simulink model "feng_rx_ct_pack"  (R2012b)
settings: Solver=FixedStepDiscrete  SolverMode=SingleTasking  StartTime=0.0  StopTime=30000  FixedStep=1  RelTol=1e-3
libraries: xbsIndex_r4 x1581, xps_library x3, casper_library_delays x2
(part 2 of 11)

== system feng_rx_ct_pack/gap_enforcer ==
  sync : Inport
  din : Inport  Port=2
  en : Inport  Port=3
  Concat : xbsIndex_r4/Concat  num_inputs=2  dbl_ovrd=off  block_type=concat
  Delay : xbsIndex_r4/Delay  rst=off  infoeditControl=Selection of Reset will increase slice count due to use of real FFs and instead of SRLs  en=off  latency=1  dbl_ovrd=off  reg_retiming=off  block_type=delay
  FIFO : xbsIndex_r4/FIFO  mem_type=Distributed RAM  performance_options=Standard_FIFO  infoedit1=Available only for V4, V5, V6, V7, K7, A7 and Zynq devices.  embedded_registers=off  depth=16  percent_nbits=2  rst=off  en=off  use_dcount=off  use_percent_full_port=off  use_almost_empty=off  almost_empty_thresh=2  use_almost_full=off  almost_full_thresh=14  dbl_ovrd=off  explicit_period=off  block_type=fifo
  Gateway Out{,1..7} (8 alike) : xbsIndex_r4/Gateway Out  inherit_from_input=off  hdl_port=on  timing_constraint=None  locs_specified=off  LOCs={}  UseAsDAC=off  DACChannel='1'  block_type=gatewayout
  Inverter : xbsIndex_r4/Inverter  en=off  latency=0  dbl_ovrd=off  block_type=inv
  Logical : xbsIndex_r4/Logical  logical_function=AND  inputs=2  en=off  latency=0  precision=Full  arith_type=Unsigned  n_bits=16  bin_pt=0  align_bp=on  dbl_ovrd=off  block_type=logical
  Scope : Scope  NumInputPorts=8
      settings: YMin=0~0~0~0~0~-1~0~-1  YMax=1~1~1~150~1~1~300~1
  Slice2 : xbsIndex_r4/Slice  nbits=1  boolean_output=off  mode=Two Bit Locations  bit1=-1  base1=MSB of Input  bit0=0  base0=LSB of Input  dbl_ovrd=off  block_type=slice
  Slice3 : xbsIndex_r4/Slice  nbits=1  boolean_output=on  mode=Upper Bit Location + Width  bit1=0  base1=MSB of Input  bit0=0  base0=LSB of Input  dbl_ovrd=off  block_type=slice
  Terminator1 : Terminator
  block_size : xbsIndex_r4/Constant  const=block_size  gui_display_data_type=Fixed-point  arith_type=Unsigned  n_bits=ceil(log2(block_size+gap_size))  bin_pt=0  preci_type=Single  exp_width=8  frac_width=24  explicit_period=on  period=1  equ=P=C  opselect=C  inp2=PCIN>>17  opr=+  inp1=P  carry=CIN  dbl_ovrd=off  block_type=constant
  data_count : xbsIndex_r4/Counter  cnt_type=Count Limited  cnt_to=block_size + gap_size  operation=Up  start_count=0  cnt_by_val=1  arith_type=Unsigned  n_bits=ceil(log2(block_size + gap_size))  bin_pt=0  load_pin=off  rst=on  en=on  explicit_period=on  period=1  dbl_ovrd=off  use_behavioral_HDL=off  implementation=Fabric  block_type=counter
  edge_detect1 : Subsystem  AncestorBlock=casper_library_misc/edge_detect  mask(edge_detect){edge=Rising, polarity=Active High, x_in=[0 0.08 0.08 0.16 0.16 0.24 0.24 0.32 0.32 0.4], y_in=[-1 -1  1  1  1  1  1  1  1  1], x_out=[0.6 0.68 0.68 0.76 0.76 0.84 0.84 0.92 0.92 1], y_out=[-1 -1  1  1 -1 -1 -1 -1 -1 -1]}
      mask prompts: edge "Edge Type"; polarity "Output Polarity"; x_in "Input X Positions"; y_in "Input Y Positions"; x_out "Output X Positions"; y_out "Output Y Positions"
      mask help: Output is active for one-cycle after each edge of the specified type (i.e. rising, falling or both).
      mask init:
      | edge_detect_init(gcb,...
      |     'edge',edge,...
      |     'polarity',polarity,...
      |     'x_in',x_in,...
      |     'x_out',x_out,...
      |     'y_in',y_in,...
      |     'y_out',y_out);
      | 
      | x_in_num=str2num(getfield(getfield(get_param(gcb,'UserData'),'parameters'),'x_in'));
      | x_out_num=str2num(getfield(getfield(get_param(gcb,'UserData'),'parameters'),'x_out'));
      | y_in_num=str2num(getfield(getfield(get_param(gcb,'UserData'),'parameters'),'y_in'));
      | y_out_num=str2num(getfield(getfield(get_param(gcb,'UserData'),'parameters'),'y_out'));
      settings: AttributesFormatString=|
      | rising edges
      | active high
      mask Help: Output is active for one-cycle after each edge of the specified type (i.e. rising, falling, or both).  Latency is zero.
      mask TypeOptions edge: Rising | Falling | Both
      mask TypeOptions polarity: Active High | Active Low
      mask Display:
      | plot(x_in_num,0.5+y_in_num*0.2);
      | plot(x_out_num,0.5+y_out_num*0.2);
  post_gap : xbsIndex_r4/Relational  mode=a<b  en=off  latency=0  dbl_ovrd=off  block_type=relational
  sync_out : Outport
  dout : Outport  Port=2
  dvalid : Outport  Port=3
  wires:
  edge_detect1/1(out) -> sync_out/1, Gateway Out5/1, data_count/1
  Logical/1 -> FIFO/3, Delay/1
  FIFO/2 -> Inverter/1
  FIFO/3 -> Terminator1/1
  post_gap/1 -> Gateway Out4/1, Logical/1
  Slice2/1 -> dout/1, Gateway Out6/1
  Inverter/1 -> Gateway Out2/1, data_count/2, Logical/2
  Slice3/1 -> edge_detect1/1(in)
  FIFO/1 -> Slice3/1, Slice2/1
  Concat/1 -> FIFO/1
  din/1 -> Concat/2
  Delay/1 -> dvalid/1, Gateway Out7/1
  en/1 -> FIFO/2, Gateway Out/1
  sync/1 -> Concat/1, Gateway Out1/1
  Gateway Out7/1 -> Scope/8
  Gateway Out6/1 -> Scope/7
  Gateway Out2/1 -> Scope/3
  Gateway Out3/1 -> Scope/4
  Gateway Out5/1 -> Scope/6
  Gateway Out4/1 -> Scope/5
  Gateway Out/1 -> Scope/1
  Gateway Out1/1 -> Scope/2
  block_size/1 -> post_gap/2
  data_count/1 -> Gateway Out3/1, post_gap/1

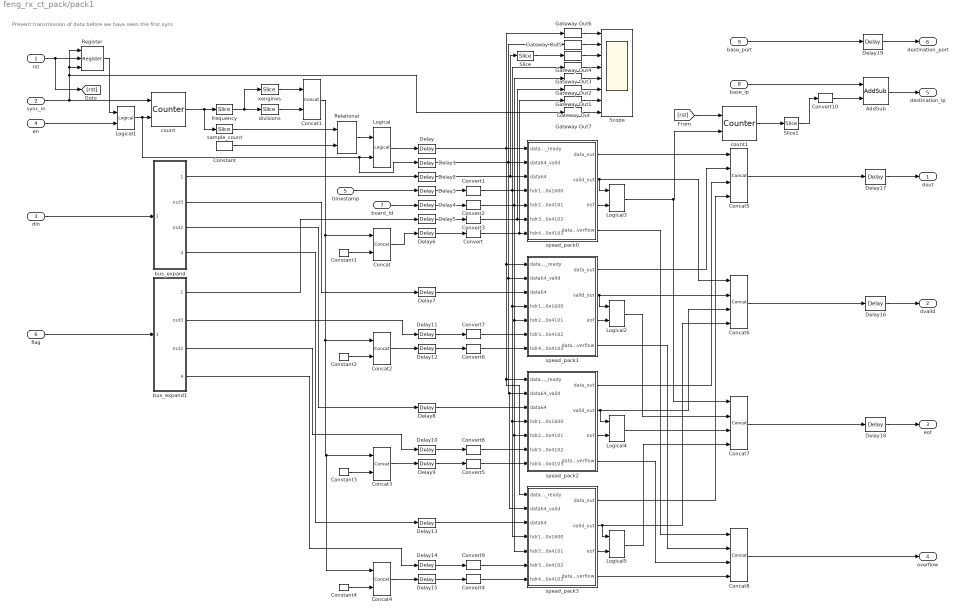
== system feng_rx_ct_pack/pack1 ==
  note: Prevent transmission of data
      | before we have seen the first
      | sync
  rst : Inport
  sync_in : Inport  Port=2
  din : Inport  Port=3
  en : Inport  Port=4
  timestamp : Inport  Port=5
  flag : Inport  Port=6
  board_id : Inport  Port=7
  base_ip : Inport  Port=8
  base_port : Inport  Port=9
  AddSub : xbsIndex_r4/AddSub  mode=Addition  use_carryin=off  use_carryout=off  en=off  latency=1  precision=User Defined  arith_type=Unsigned  n_bits=32  bin_pt=0  quantization=Truncate  overflow=Wrap  dbl_ovrd=off  use_behavioral_HDL=off  hw_selection=Fabric  pipelined=off  block_type=addsub
  Concat{,1..4} (5 alike) : xbsIndex_r4/Concat  num_inputs=2  dbl_ovrd=off  block_type=concat
  Concat{5..8} (4 alike) : xbsIndex_r4/Concat  num_inputs=4  dbl_ovrd=off  block_type=concat
  Constant : xbsIndex_r4/Constant  const=0  gui_display_data_type=Fixed-point  arith_type=Unsigned  n_bits=n_bits_packet - n_bits_inputs  bin_pt=0  preci_type=Single  exp_width=8  frac_width=24  explicit_period=on  period=1  equ=P=C  opselect=C  inp2=PCIN>>17  opr=+  inp1=P  carry=CIN  dbl_ovrd=off  block_type=constant
  Constant1 : xbsIndex_r4/Constant  const=0  gui_display_data_type=Fixed-point  arith_type=Unsigned  n_bits=2  bin_pt=0  preci_type=Single  exp_width=8  frac_width=24  explicit_period=on  period=1  equ=P=C  opselect=C  inp2=PCIN>>17  opr=+  inp1=P  carry=CIN  dbl_ovrd=off  block_type=constant
  Constant2 : xbsIndex_r4/Constant  const=1  gui_display_data_type=Fixed-point  arith_type=Unsigned  n_bits=2  bin_pt=0  preci_type=Single  exp_width=8  frac_width=24  explicit_period=on  period=1  equ=P=C  opselect=C  inp2=PCIN>>17  opr=+  inp1=P  carry=CIN  dbl_ovrd=off  block_type=constant
  Constant3 : xbsIndex_r4/Constant  const=2  gui_display_data_type=Fixed-point  arith_type=Unsigned  n_bits=2  bin_pt=0  preci_type=Single  exp_width=8  frac_width=24  explicit_period=on  period=1  equ=P=C  opselect=C  inp2=PCIN>>17  opr=+  inp1=P  carry=CIN  dbl_ovrd=off  block_type=constant
  Constant4 : xbsIndex_r4/Constant  const=3  gui_display_data_type=Fixed-point  arith_type=Unsigned  n_bits=2  bin_pt=0  preci_type=Single  exp_width=8  frac_width=24  explicit_period=on  period=1  equ=P=C  opselect=C  inp2=PCIN>>17  opr=+  inp1=P  carry=CIN  dbl_ovrd=off  block_type=constant
  Convert{,1..9} (10 alike) : xbsIndex_r4/Convert  gui_display_data_type=Fixed-point  arith_type=Unsigned  n_bits=48  bin_pt=0  float_type=Single  exp_bits=8  fraction_bits=24  quantization=Truncate  overflow=Wrap  en=off  latency=0  dbl_ovrd=off  pipeline=off  block_type=convert
  Convert10 : xbsIndex_r4/Convert  gui_display_data_type=Fixed-point  arith_type=Unsigned  n_bits=32  bin_pt=0  float_type=Single  exp_bits=8  fraction_bits=24  quantization=Truncate  overflow=Wrap  en=off  latency=0  dbl_ovrd=off  pipeline=off  block_type=convert
  Delay{,16..19} (5 alike) : xbsIndex_r4/Delay  rst=off  infoeditControl=Selection of Reset will increase slice count due to use of real FFs and instead of SRLs  en=off  latency=1  dbl_ovrd=off  reg_retiming=on  block_type=delay
  Delay{1..15} (15 alike) : xbsIndex_r4/Delay  rst=off  infoeditControl=Selection of Reset will increase slice count due to use of real FFs and instead of SRLs  en=off  latency=2  dbl_ovrd=off  reg_retiming=on  block_type=delay
  Gateway Out{,1..7} (8 alike) : xbsIndex_r4/Gateway Out  inherit_from_input=off  hdl_port=on  timing_constraint=None  locs_specified=off  LOCs={}  UseAsDAC=off  DACChannel='1'  block_type=gatewayout
  Logical{,1..5} (6 alike) : xbsIndex_r4/Logical  logical_function=AND  inputs=2  en=off  latency=0  precision=Full  arith_type=Unsigned  n_bits=16  bin_pt=0  align_bp=on  dbl_ovrd=off  block_type=logical
  Register : xbsIndex_r4/Register  init=0  rst=on  en=on  dbl_ovrd=off  block_type=register
  Relational : xbsIndex_r4/Relational  mode=a=b  en=off  latency=0  dbl_ovrd=off  block_type=relational
  Scope : Scope  NumInputPorts=8
      settings: YMin=-1~-1~832.2~3.11296e+06~-1~-1~26.6~-1  YMax=1~1~919.8~3.44064e+06~1~1~29.4~1  SaveName=ScopeData11
  Slice : xbsIndex_r4/Slice  nbits=16  boolean_output=off  mode=Upper Bit Location + Width  bit1=0  base1=MSB of Input  bit0=0  base0=LSB of Input  dbl_ovrd=off  block_type=slice
  Slice1 : xbsIndex_r4/Slice  nbits=n_bits_xengines - n_bits_xeng_per_ip  boolean_output=off  mode=Upper Bit Location + Width  bit1=0  base1=MSB of Input  bit0=0  base0=LSB of Input  dbl_ovrd=off  block_type=slice
  bus_expand : Subsystem  AncestorBlock=casper_library_flow_control/bus_expand  mask(bus_expand){mode=divisions of equal size, outputNum=4, outputWidth=64, outputBinaryPt=0, outputArithmeticType=0, show_format=off, outputToWorkspace=off, variablePrefix=out, outputToModelAsWell=on}
      mask prompts: outputNum "Number of outputs:"; outputWidth "Output width:"; outputBinaryPt "Output binary point position:"; outputArithmeticType "Output arithmetic type (ufix=0, fix=1, bool=2):"; show_format "Print format string?"; outputToWorkspace "Output to workspace?"; variablePrefix "Variable name prefix:"; outputToModelAsWell "Output to model as well?"
      mask help:
      | Expands a 'bus' made using a bus_create or Xilinx
      | concat block.
      | The input will be divided into the specified number
      | of outputs with the specified arithmetic types.
      | Divisions are made from most significant bit.
      mask init: same as feng_rx_ct_pack/bus_expand11
      settings: AttributesFormatString=4 outputs
      mask TypeOptions mode: divisions of equal size | divisions of arbitrary size
      mask Callback mode: bus_expand_callback();
      mask Callback outputWidth: bus_expand_callback();
      mask Callback outputToWorkspace: bus_expand_callback();
  bus_expand1 : Subsystem  AncestorBlock=casper_library_flow_control/bus_expand  mask(bus_expand){mode=divisions of equal size, outputNum=4, outputWidth=1, outputBinaryPt=0, outputArithmeticType=0, show_format=off, outputToWorkspace=off, variablePrefix=out, outputToModelAsWell=on}
      mask prompts: outputNum "Number of outputs:"; outputWidth "Output width:"; outputBinaryPt "Output binary point position:"; outputArithmeticType "Output arithmetic type (ufix=0, fix=1, bool=2):"; show_format "Print format string?"; outputToWorkspace "Output to workspace?"; variablePrefix "Variable name prefix:"; outputToModelAsWell "Output to model as well?"
      mask help:
      | Expands a 'bus' made using a bus_create or Xilinx
      | concat block.
      | The input will be divided into the specified number
      | of outputs with the specified arithmetic types.
      | Divisions are made from most significant bit.
      mask init: same as feng_rx_ct_pack/bus_expand11
      settings: AttributesFormatString=4 outputs
      mask TypeOptions mode: divisions of equal size | divisions of arbitrary size
      mask Callback mode: bus_expand_callback();
      mask Callback outputWidth: bus_expand_callback();
      mask Callback outputToWorkspace: bus_expand_callback();
  count : xbsIndex_r4/Counter  cnt_type=Free Running  cnt_to=Inf  operation=Up  start_count=0  cnt_by_val=1  arith_type=Unsigned  n_bits=n_bits_frequencies + n_bits_packet - n_bits_inputs  bin_pt=0  load_pin=off  rst=on  en=on  explicit_period=on  period=1  dbl_ovrd=off  use_behavioral_HDL=off  implementation=Fabric  block_type=counter
  count1 : xbsIndex_r4/Counter  cnt_type=Free Running  cnt_to=Inf  operation=Up  start_count=0  cnt_by_val=1  arith_type=Unsigned  n_bits=n_bits_xengines  bin_pt=0  load_pin=off  rst=on  en=on  explicit_period=on  period=1  dbl_ovrd=off  use_behavioral_HDL=off  implementation=Fabric  block_type=counter
  divisions : xbsIndex_r4/Slice  nbits=n_bits_frequencies - n_bits_xengines  boolean_output=off  mode=Upper Bit Location + Width  bit1=0  base1=MSB of Input  bit0=0  base0=LSB of Input  dbl_ovrd=off  block_type=slice
  frequency : xbsIndex_r4/Slice  nbits=n_bits_frequencies  boolean_output=off  mode=Upper Bit Location + Width  bit1=0  base1=MSB of Input  bit0=0  base0=LSB of Input  dbl_ovrd=off  block_type=slice
  sample_count : xbsIndex_r4/Slice  nbits=n_bits_packet - n_bits_inputs  boolean_output=off  mode=Lower Bit Location + Width  bit1=0  base1=MSB of Input  bit0=0  base0=LSB of Input  dbl_ovrd=off  block_type=slice
  spead_pack0 : Subsystem  Tag=casper:spead_pack  AncestorBlock=casper_library_communications/spead_pack  mask(pkt_pack_mask){payload_length=2^(n_bits_packet - n_bits_inputs), header_ids=hex2dec({'1600', '4101', '4102', '4103'}), spead_msw=64, spead_lsw=48, spead_version=4}
      mask prompts: payload_length "Payload Length in 64-bit words"; header_ids "SPEAD header IDs (decimal)"; spead_msw "SPEAD Flavour (MSw)"; spead_lsw "SPEAD Flavour (LSw)"; spead_version "SPEAD version"
      mask help:
      | This block generates SPEAD-compliant packets from a datastream.
      |
      | Packets are created with a fixed header followed by a number of 64-bit items.
      |
      | Requires a 64-bit data stream.
      |
      | See the documentation for further details.
      mask init:
      | spead_pack_init(gcb, header_ids)
  spead_pack1 : Subsystem  Tag=casper:spead_pack  AncestorBlock=casper_library_communications/spead_pack  mask(pkt_pack_mask){payload_length=2^(n_bits_packet - n_bits_inputs), header_ids=hex2dec({'1600', '4101', '4102', '4103'}), spead_msw=64, spead_lsw=48, spead_version=4}
      mask prompts: payload_length "Payload Length in 64-bit words"; header_ids "SPEAD header IDs (decimal)"; spead_msw "SPEAD Flavour (MSw)"; spead_lsw "SPEAD Flavour (LSw)"; spead_version "SPEAD version"
      mask help:
      | This block generates SPEAD-compliant packets from a datastream.
      |
      | Packets are created with a fixed header followed by a number of 64-bit items.
      |
      | Requires a 64-bit data stream.
      |
      | See the documentation for further details.
      mask init:
      | spead_pack_init(gcb, header_ids)
  spead_pack2 : Subsystem  Tag=casper:spead_pack  AncestorBlock=casper_library_communications/spead_pack  mask(pkt_pack_mask){payload_length=2^(n_bits_packet - n_bits_inputs), header_ids=hex2dec({'1600', '4101', '4102', '4103'}), spead_msw=64, spead_lsw=48, spead_version=4}
      mask prompts: payload_length "Payload Length in 64-bit words"; header_ids "SPEAD header IDs (decimal)"; spead_msw "SPEAD Flavour (MSw)"; spead_lsw "SPEAD Flavour (LSw)"; spead_version "SPEAD version"
      mask help:
      | This block generates SPEAD-compliant packets from a datastream.
      |
      | Packets are created with a fixed header followed by a number of 64-bit items.
      |
      | Requires a 64-bit data stream.
      |
      | See the documentation for further details.
      mask init:
      | spead_pack_init(gcb, header_ids)
  spead_pack3 : Subsystem  Tag=casper:spead_pack  AncestorBlock=casper_library_communications/spead_pack  mask(pkt_pack_mask){payload_length=2^(n_bits_packet - n_bits_inputs), header_ids=hex2dec({'1600', '4101', '4102', '4103'}), spead_msw=64, spead_lsw=48, spead_version=4}
      mask prompts: payload_length "Payload Length in 64-bit words"; header_ids "SPEAD header IDs (decimal)"; spead_msw "SPEAD Flavour (MSw)"; spead_lsw "SPEAD Flavour (LSw)"; spead_version "SPEAD version"
      mask help:
      | This block generates SPEAD-compliant packets from a datastream.
      |
      | Packets are created with a fixed header followed by a number of 64-bit items.
      |
      | Requires a 64-bit data stream.
      |
      | See the documentation for further details.
      mask init:
      | spead_pack_init(gcb, header_ids)
  xengines : xbsIndex_r4/Slice  nbits=n_bits_xengines  boolean_output=off  mode=Lower Bit Location + Width  bit1=0  base1=MSB of Input  bit0=0  base0=LSB of Input  dbl_ovrd=off  block_type=slice
  dout : Outport
  dvalid : Outport  Port=2
  eof : Outport  Port=3
  overflow : Outport  Port=4
  destination_ip : Outport  Port=5
  destination_port : Outport  Port=6
  wires:
  Logical5/1 -> Concat7/4
  spead_pack3/3(eof) -> Logical5/2
  Logical4/1 -> Concat7/3
  spead_pack2/3(eof) -> Logical4/2
  Logical3/1 -> count1/2, Concat7/1
  spead_pack0/3(eof) -> Logical3/2
  Logical2/1 -> Concat7/2
  spead_pack1/3(eof) -> Logical2/2
  Slice1/1 -> Convert10/1
  Convert10/1 -> AddSub/2
  AddSub/1 -> destination_ip/1
  count1/1 -> Slice1/1
  Delay19/1 -> destination_port/1
  base_port/1 -> Delay19/1
  Delay18/1 -> eof/1
  Delay16/1 -> dvalid/1
  Delay17/1 -> dout/1
  base_ip/1 -> AddSub/1
  [rst] -> count1/1
  Convert9/1 -> spead_pack3/6(hdr3_0x4102)
  Convert8/1 -> spead_pack2/6(hdr3_0x4102)
  Convert7/1 -> spead_pack1/6(hdr3_0x4102)
  Convert6/1 -> spead_pack1/7(hdr4_0x4103)
  Convert5/1 -> spead_pack2/7(hdr4_0x4103)
  Convert4/1 -> spead_pack3/7(hdr4_0x4103)
  Concat8/1 -> overflow/1
  Concat7/1 -> Delay18/1
  Concat6/1 -> Delay16/1
  spead_pack3/4(data_overflow) -> Concat8/4
  spead_pack2/4(data_overflow) -> Concat8/3
  spead_pack1/4(data_overflow) -> Concat8/2
  spead_pack0/4(data_overflow) -> Concat8/1
  spead_pack3/2(valid_out) -> Concat6/4, Logical5/1
  spead_pack2/2(valid_out) -> Concat6/3, Logical4/1
  spead_pack1/2(valid_out) -> Concat6/2, Logical2/1
  spead_pack0/2(valid_out) -> Logical3/1, Concat6/1
  Concat5/1 -> Delay17/1
  spead_pack3/1(data_out) -> Concat5/4
  spead_pack2/1(data_out) -> Concat5/3
  spead_pack1/1(data_out) -> Concat5/2
  spead_pack0/1(data_out) -> Concat5/1
  Concat4/1 -> Delay15/1
  Delay15/1 -> Convert4/1
  Constant4/1 -> Concat4/2
  bus_expand1/4(lsb_out1) -> Delay14/1
  Delay14/1 -> Convert9/1
  Delay13/1 -> spead_pack3/3(data64)
  bus_expand/4(lsb_out1) -> Delay13/1
  Delay9/1 -> Convert5/1
  Concat3/1 -> Delay9/1
  Constant3/1 -> Concat3/2
  Delay10/1 -> Convert8/1
  bus_expand1/3(out2) -> Delay10/1
  Delay12/1 -> Convert6/1
  Delay11/1 -> Convert7/1
  bus_expand1/2(out3) -> Delay11/1
  Delay8/1 -> spead_pack2/3(data64)
  bus_expand/3(out2) -> Delay8/1
  Concat2/1 -> Delay12/1
  Delay7/1 -> spead_pack1/3(data64)
  bus_expand/2(out3) -> Delay7/1
  Concat1/1 -> Concat2/1, Concat3/1, Concat4/1, Concat/1
  Constant2/1 -> Concat2/2
  bus_expand1/1(msb_out4) -> Delay5/1
  flag/1 -> bus_expand1/1(bus_in)
  divisions/1 -> Concat1/2
  xengines/1 -> Concat1/1
  frequency/1 -> xengines/1, divisions/1
  Slice/1 -> Gateway Out4/1
  Concat/1 -> Delay6/1
  Constant1/1 -> Concat/2
  Logical1/1 -> count/2, Logical/2, Delay1/1
  en/1 -> Logical1/2
  Register/1 -> Logical1/1
  rst/1 -> Register/2, [rst]
  sync_in/1 -> Gateway Out7/1, Register/3, Register/1, count/1
  Gateway Out7/1 -> Scope/8
  Gateway Out6/1 -> Scope/1
  Gateway Out5/1 -> Scope/2
  Gateway Out4/1 -> Scope/3
  Gateway Out3/1 -> Scope/4
  Gateway Out2/1 -> Scope/5
  Gateway Out1/1 -> Scope/6
  Gateway Out/1 -> Scope/7
  Delay2/1 -> Slice/1, spead_pack0/3(data64)
  Delay6/1 -> Convert/1
  Delay5/1 -> Convert3/1
  Delay4/1 -> Convert2/1
  Delay3/1 -> Convert1/1
  Delay1/1 -> Gateway Out5/1, spead_pack3/2(data64_valid), spead_pack2/2(data64_valid), spead_pack1/2(data64_valid), spead_pack0/2(data64_valid)
  Delay/1 -> Gateway Out6/1, spead_pack2/1(data64_ready), spead_pack3/1(data64_ready), spead_pack1/1(data64_ready), spead_pack0/1(data64_ready)
  Logical/1 -> Delay/1
  Relational/1 -> Logical/1
  Constant/1 -> Relational/2
  sample_count/1 -> Relational/1
  bus_expand/1(msb_out4) -> Delay2/1
  din/1 -> bus_expand/1(bus_in)
  board_id/1 -> Delay4/1
  Convert3/1 -> Gateway Out1/1, spead_pack0/6(hdr3_0x4102)
  Convert2/1 -> Gateway Out2/1, spead_pack2/5(hdr2_0x4101), spead_pack3/5(hdr2_0x4101), spead_pack1/5(hdr2_0x4101), spead_pack0/5(hdr2_0x4101)
  Convert1/1 -> Gateway Out3/1, spead_pack3/4(hdr1_0x1600), spead_pack2/4(hdr1_0x1600), spead_pack1/4(hdr1_0x1600), spead_pack0/4(hdr1_0x1600)
  timestamp/1 -> Delay3/1
  Convert/1 -> Gateway Out/1, spead_pack0/7(hdr4_0x4103)
  count/1 -> frequency/1, sample_count/1

== system feng_rx_ct_pack/sync_gen1 ==
  note: generate single sync pulse
      | on first block edge after
      | a reset or an error
  note: generate sync
      | on last sample of
      | data block
  note: check that 0 timestamps
      | are the correct number of data
      | samples apart
  rst : Inport
  din : Inport  Port=2
  en : Inport  Port=3
  time_in : Inport  Port=4
  Gateway Out{1..10} (10 alike) : xbsIndex_r4/Gateway Out  inherit_from_input=off  hdl_port=on  timing_constraint=None  locs_specified=off  LOCs={}  UseAsDAC=off  DACChannel='1'  block_type=gatewayout
  Logical1 : xbsIndex_r4/Logical  logical_function=XOR  inputs=2  en=off  latency=0  precision=Full  arith_type=Unsigned  n_bits=16  bin_pt=0  align_bp=on  dbl_ovrd=off  block_type=logical
  Logical2 : xbsIndex_r4/Logical  logical_function=OR  inputs=2  en=off  latency=0  precision=Full  arith_type=Unsigned  n_bits=16  bin_pt=0  align_bp=on  dbl_ovrd=off  block_type=logical
  Logical{3..6} (4 alike) : xbsIndex_r4/Logical  logical_function=AND  inputs=2  en=off  latency=0  precision=Full  arith_type=Unsigned  n_bits=16  bin_pt=0  align_bp=on  dbl_ovrd=off  block_type=logical
  Relational : xbsIndex_r4/Relational  mode=a=b  en=off  latency=1  dbl_ovrd=off  block_type=relational
  Relational1 : xbsIndex_r4/Relational  mode=a=b  en=off  latency=0  dbl_ovrd=off  block_type=relational
  Relational3 : xbsIndex_r4/Relational  mode=a=b  en=off  latency=0  dbl_ovrd=off  block_type=relational
  Scope1 : Scope  NumInputPorts=7
      settings: YMin=1.525e+06~-1~-1~-1~1.525e+06~-5~-5  YMax=1.565e+06~1~1~1~1.565e+06~5~5  SaveName=ScopeData3
  Scope2 : Scope  NumInputPorts=3
      settings: YMin=1~0~0  YMax=1~1~1  SaveName=ScopeData4
  constant : xbsIndex_r4/Constant  const=0  gui_display_data_type=Fixed-point  arith_type=Unsigned  n_bits=(n_bits_frequencies - n_bits_streams) + n_bits_packet_size + 1  bin_pt=0  preci_type=Single  exp_width=8  frac_width=24  explicit_period=on  period=1  equ=P=C  opselect=C  inp2=PCIN>>17  opr=+  inp1=P  carry=CIN  dbl_ovrd=off  block_type=constant
  constant1 : xbsIndex_r4/Constant  const=0  gui_display_data_type=Fixed-point  arith_type=Unsigned  n_bits=(n_bits_frequencies - n_bits_streams) + n_bits_packet_size + 1  bin_pt=0  preci_type=Single  exp_width=8  frac_width=24  explicit_period=on  period=1  equ=P=C  opselect=C  inp2=PCIN>>17  opr=+  inp1=P  carry=CIN  dbl_ovrd=off  block_type=constant
  counter : xbsIndex_r4/Counter  cnt_type=Count Limited  cnt_to=2^((n_bits_frequencies - n_bits_streams) + n_bits_packet_size + 1 + n_bits_count) * (reorder_order*unscrambler_order) - 2^n_bits_count  operation=Up  start_count=0  cnt_by_val=2^n_bits_count  arith_type=Unsigned  n_bits=(n_bits_frequencies - n_bits_streams) + n_bits_packet_size + 1 + ceil(log2(reorder_order*unscrambler_order)) + n_bits_count  bin_pt=0  load_pin=off  rst=on  en=on  explicit_period=on  period=1  dbl_ovrd=off  use_behavioral_HDL=off  implementation=Fabric  block_type=counter
  ddin{0..2,4} (4 alike) : xbsIndex_r4/Delay  rst=off  infoeditControl=Selection of Reset will increase slice count due to use of real FFs and instead of SRLs  en=off  latency=1  dbl_ovrd=off  reg_retiming=on  block_type=delay
  ddin3 : xbsIndex_r4/Delay  rst=off  infoeditControl=Selection of Reset will increase slice count due to use of real FFs and instead of SRLs  en=on  latency=2  dbl_ovrd=off  reg_retiming=on  block_type=delay
  dedge0 : xbsIndex_r4/Delay  rst=off  infoeditControl=Selection of Reset will increase slice count due to use of real FFs and instead of SRLs  en=off  latency=1  dbl_ovrd=off  reg_retiming=on  block_type=delay
  dedge1 : xbsIndex_r4/Delay  rst=off  infoeditControl=Selection of Reset will increase slice count due to use of real FFs and instead of SRLs  en=off  latency=1  dbl_ovrd=off  reg_retiming=on  block_type=delay
  dedge2 : xbsIndex_r4/Delay  rst=on  infoeditControl=Selection of Reset will increase slice count due to use of real FFs and instead of SRLs  en=on  latency=1  dbl_ovrd=off  reg_retiming=off  block_type=delay
  den{0..4} (5 alike) : xbsIndex_r4/Delay  rst=off  infoeditControl=Selection of Reset will increase slice count due to use of real FFs and instead of SRLs  en=off  latency=1  dbl_ovrd=off  reg_retiming=on  block_type=delay
  derr : xbsIndex_r4/Delay  rst=off  infoeditControl=Selection of Reset will increase slice count due to use of real FFs and instead of SRLs  en=off  latency=1  dbl_ovrd=off  reg_retiming=on  block_type=delay
  dsync : xbsIndex_r4/Delay  rst=off  infoeditControl=Selection of Reset will increase slice count due to use of real FFs and instead of SRLs  en=off  latency=1  dbl_ovrd=off  reg_retiming=on  block_type=delay
  dtime{0..2,4} (4 alike) : xbsIndex_r4/Delay  rst=off  infoeditControl=Selection of Reset will increase slice count due to use of real FFs and instead of SRLs  en=off  latency=1  dbl_ovrd=off  reg_retiming=on  block_type=delay
  dtime3 : xbsIndex_r4/Delay  rst=off  infoeditControl=Selection of Reset will increase slice count due to use of real FFs and instead of SRLs  en=on  latency=2  dbl_ovrd=off  reg_retiming=on  block_type=delay
  edge_detect : Subsystem  AncestorBlock=casper_library_misc/edge_detect  mask(edge_detect){edge=Rising, polarity=Active High, x_in=[0 0.08 0.08 0.16 0.16 0.24 0.24 0.32 0.32 0.4], y_in=[-1 -1  1  1  1  1  1  1  1  1], x_out=[0.6 0.68 0.68 0.76 0.76 0.84 0.84 0.92 0.92 1], y_out=[-1 -1  1  1 -1 -1 -1 -1 -1 -1]}
      mask prompts: edge "Edge Type"; polarity "Output Polarity"; x_in "Input X Positions"; y_in "Input Y Positions"; x_out "Output X Positions"; y_out "Output Y Positions"
      mask help: Output is active for one-cycle after each edge of the specified type (i.e. rising, falling or both).
      mask init: same as feng_rx_ct_pack/gap_enforcer/edge_detect1
      settings: AttributesFormatString=|
      | rising edges
      | active high
      mask Help: Output is active for one-cycle after each edge of the specified type (i.e. rising, falling, or both).  Latency is zero.
      mask TypeOptions edge: Rising | Falling | Both
      mask TypeOptions polarity: Active High | Active Low
      mask Display:
      | plot(x_in_num,0.5+y_in_num*0.2);
      | plot(x_out_num,0.5+y_out_num*0.2);
  edge_detect1 : Subsystem  AncestorBlock=casper_library_misc/edge_detect  mask(edge_detect){edge=Rising, polarity=Active High, x_in=[0 0.08 0.08 0.16 0.16 0.24 0.24 0.32 0.32 0.4], y_in=[-1 -1  1  1  1  1  1  1  1  1], x_out=[0.6 0.68 0.68 0.76 0.76 0.84 0.84 0.92 0.92 1], y_out=[-1 -1  1  1 -1 -1 -1 -1 -1 -1]}
      mask prompts: edge "Edge Type"; polarity "Output Polarity"; x_in "Input X Positions"; y_in "Input Y Positions"; x_out "Output X Positions"; y_out "Output Y Positions"
      mask help: Output is active for one-cycle after each edge of the specified type (i.e. rising, falling or both).
      mask init: same as feng_rx_ct_pack/gap_enforcer/edge_detect1
      settings: AttributesFormatString=|
      | rising edges
      | active high
      mask Help: Output is active for one-cycle after each edge of the specified type (i.e. rising, falling, or both).  Latency is zero.
      mask TypeOptions edge: Rising | Falling | Both
      mask TypeOptions polarity: Active High | Active Low
      mask Display:
      | plot(x_in_num,0.5+y_in_num*0.2);
      | plot(x_out_num,0.5+y_out_num*0.2);
  first : xbsIndex_r4/Delay  rst=on  infoeditControl=Selection of Reset will increase slice count due to use of real FFs and instead of SRLs  en=on  latency=1  dbl_ovrd=off  reg_retiming=on  block_type=delay
  locked : xbsIndex_r4/Delay  rst=off  infoeditControl=Selection of Reset will increase slice count due to use of real FFs and instead of SRLs  en=on  latency=1  dbl_ovrd=off  reg_retiming=on  block_type=delay
  lsbs_count : xbsIndex_r4/Slice  nbits=(n_bits_frequencies - n_bits_streams) + n_bits_packet_size + 1  boolean_output=off  mode=Lower Bit Location + Width  bit1=0  base1=MSB of Input  bit0=0  base0=LSB of Input  dbl_ovrd=off  block_type=slice
  lsbs_timestamp : xbsIndex_r4/Slice  nbits=(n_bits_frequencies - n_bits_streams) + n_bits_packet_size + 1  boolean_output=off  mode=Lower Bit Location + Width  bit1=0  base1=MSB of Input  bit0=0  base0=LSB of Input  dbl_ovrd=off  block_type=slice
  sample_count : xbsIndex_r4/Constant  const=0  gui_display_data_type=Fixed-point  arith_type=Unsigned  n_bits=(n_bits_frequencies - n_bits_streams) + n_bits_packet_size + 1 + ceil(log2(reorder_order*unscrambler_order)) + n_bits_count  bin_pt=0  preci_type=Single  exp_width=8  frac_width=24  explicit_period=on  period=1  equ=P=C  opselect=C  inp2=PCIN>>17  opr=+  inp1=P  carry=CIN  dbl_ovrd=off  block_type=constant
  sync : Outport
  dout : Outport  Port=2
  dvalid : Outport  Port=3
  time_out : Outport  Port=4
  error : Outport  Port=5
  wires:
  edge_detect1/1(out) -> dedge0/1
  Gateway Out2/1 -> Scope1/7
  Gateway Out10/1 -> Scope1/6
  dedge0/1 -> Gateway Out7/1, locked/2, dedge1/1
  Relational/1 -> edge_detect1/1(in)
  dtime4/1 -> dtime1/1
  den4/1 -> den1/1
  ddin4/1 -> ddin1/1
  dsync/1 -> sync/1
  dedge1/1 -> dedge2/3, dedge2/1
  dtime1/1 -> dtime2/1
  ddin1/1 -> ddin2/1
  den1/1 -> den2/1
  den2/1 -> counter/2, Logical5/2, Logical6/1, Logical3/2, den3/1, dtime3/2, ddin3/2, Gateway Out10/1
  ddin2/1 -> ddin3/1, Gateway Out2/1
  dtime2/1 -> Gateway Out1/1, dtime3/1
  den0/1 -> den4/1
  Logical3/1 -> dsync/1
  Logical5/1 -> dedge2/2, Gateway Out5/1, Logical1/2
  Logical6/1 -> Gateway Out4/1, Logical1/1
  Gateway Out1/1 -> Scope1/5
  dedge2/1 -> Logical5/1
  Relational3/1 -> Logical6/2
  lsbs_timestamp/1 -> Relational/1
  Gateway Out9/1 -> Scope1/4
  Logical4/1 -> first/2
  Logical2/1 -> Logical4/2
  Gateway Out8/1 -> Scope2/3
  Gateway Out7/1 -> Scope2/2
  Gateway Out6/1 -> Scope2/1
  Gateway Out5/1 -> Scope1/3
  Gateway Out4/1 -> Scope1/2
  Gateway Out3/1 -> Scope1/1
  rst/1 -> Logical2/1
  derr/1 -> error/1
  Logical1/1 -> Logical2/2, Gateway Out9/1, derr/1
  constant1/1 -> Relational3/2
  lsbs_count/1 -> Relational3/1
  ddin3/1 -> dout/1
  den3/1 -> dvalid/1
  dtime3/1 -> time_out/1
  Relational1/1 -> Logical3/1
  counter/1 -> lsbs_count/1, Gateway Out3/1, Relational1/1
  sample_count/1 -> Relational1/2
  edge_detect/1(out) -> counter/1
  first/1 -> Gateway Out6/1, locked/1
  dtime0/1 -> dtime4/1
  ddin0/1 -> ddin4/1
  locked/1 -> Gateway Out8/1, Logical4/1, edge_detect/1(in)
  time_in/1 -> dtime0/1, lsbs_timestamp/1
  constant/1 -> Relational/2
  din/1 -> ddin0/1
  en/1 -> first/3, first/1, den0/1

== system feng_rx_ct_pack/ct1/bus_expand ==
  bus_in : Inport
  reinterpret{1..4} (4 alike) : xbsIndex_r4/Reinterpret  force_arith_type=on  arith_type=Unsigned  force_bin_pt=on  bin_pt=0  block_type=reinterpret
  slice1 : xbsIndex_r4/Slice  nbits=64  boolean_output=off  mode=Upper Bit Location + Width  bit1=-192  base1=MSB of Input  bit0=0  base0=LSB of Input  dbl_ovrd=off  block_type=slice
  slice2 : xbsIndex_r4/Slice  nbits=64  boolean_output=off  mode=Upper Bit Location + Width  bit1=-128  base1=MSB of Input  bit0=0  base0=LSB of Input  dbl_ovrd=off  block_type=slice
  slice3 : xbsIndex_r4/Slice  nbits=64  boolean_output=off  mode=Upper Bit Location + Width  bit1=-64  base1=MSB of Input  bit0=0  base0=LSB of Input  dbl_ovrd=off  block_type=slice
  slice4 : xbsIndex_r4/Slice  nbits=64  boolean_output=off  mode=Upper Bit Location + Width  bit1=0  base1=MSB of Input  bit0=0  base0=LSB of Input  dbl_ovrd=off  block_type=slice
  msb_out4 : Outport
  out3 : Outport  Port=2
  out2 : Outport  Port=3
  lsb_out1 : Outport  Port=4
  wires:
  reinterpret1/1 -> lsb_out1/1
  slice1/1 -> reinterpret1/1
  reinterpret2/1 -> out2/1
  slice2/1 -> reinterpret2/1
  reinterpret3/1 -> out3/1
  slice3/1 -> reinterpret3/1
  reinterpret4/1 -> msb_out4/1
  slice4/1 -> reinterpret4/1
  bus_in/1 -> slice1/1, slice2/1, slice3/1, slice4/1
